simulink model "mrefrobotarm_previous_y_previous_u_previous_ref_cex_3b"  (R2018b)
settings: Solver=FixedStepAuto  StartTime=0.0  StopTime=20  RelTol=1e-3  AbsTol=1e-6
undefined symbols (not defined in the file or in its folder): cc, options
libraries: neural x462, simulink x2
(part 8 of 18)

== system mrefrobotarm_previous_y_previous_u_previous_ref_cex_3b/15000 epoch/Layer 3/Delays 1 ==
  "p{3}" : Inport  PortDimensions=30
      mask Display: e = 0.06;c1 = [120 230 180]/255;c2 = ([120 230 180]+0)/(256+128);c3 = ([120 230 180]+128)/(256+128);patch([0 1 1 0],[0 0 1 1],c1);patch([0 1 1 1-e 1-e 0+e],[0 0 1 1-e 0+e 0+e],c2);patch([0 0 1 1-e 0+e 0+e],[0 1 1 1-e 1-e 0+e],c3);plot([0 1 1 0 0],[0 0 1 1 0]);
  mux : Mux  Inputs=1
      mask Display: e = 0.06;c1 = [120 150 230]/255;c2 = ([120 150 230]+0)/383;c3 = ([120 150 230]+128)/383;patch([0 1 1 0],[0 0 1 1],c1);patch([0 1 1 1-e 1-e 0+e],[0 0 1 1-e 0+e 0+e],c2);patch([0 0 1 1-e 0+e 0+e],[0 1 1 1-e 1-e 0+e],c3);plot([0 1 1 0 0],[0 0 1 1 0]);disp('Mux')
  "pd{3,2}" : Outport
      mask Display: e = 0.06;c1 = [120 230 180]/255;c2 = ([120 230 180]+0)/(256+128);c3 = ([120 230 180]+128)/(256+128);patch([0 1 1 0],[0 0 1 1],c1);patch([0 1 1 1-e 1-e 0+e],[0 0 1 1-e 0+e 0+e],c2);patch([0 0 1 1-e 0+e 0+e],[0 1 1 1-e 1-e 0+e],c3);plot([0 1 1 0 0],[0 0 1 1 0]);
  wires:
  "p{3}"/1 -> mux/1
  mux/1 -> "pd{3,2}"/1

== system mrefrobotarm_previous_y_previous_u_previous_ref_cex_3b/15000 epoch/Layer 3/LW{3,2} ==
  "ad{3,2}" : Inport  PortDimensions=30
      mask Display: e = 0.06;c1 = [120 230 180]/255;c2 = ([120 230 180]+0)/(256+128);c3 = ([120 230 180]+128)/(256+128);patch([0 1 1 0],[0 0 1 1],c1);patch([0 1 1 1-e 1-e 0+e],[0 0 1 1-e 0+e 0+e],c2);patch([0 0 1 1-e 0+e 0+e],[0 1 1 1-e 1-e 0+e],c3);plot([0 1 1 0 0],[0 0 1 1 0]);
  "IW{3,2}(1,:)'" : Constant  Value=[0.85686770362183561910995877042296342551708221435546875;0.2506520137647199053532176549197174608707427978515625;0.5892150836046241568766390628297813236713409423828125;-0.7174409906013246018829931927029974758625030517578125;-0.68953568727712888364322907364112325012683868408203125;0.69140544006949611333112670763512142002582550048828125;0.5232408762883873354354591356241144239902496337890625;-0.087728735547543623685129432487883605062961578369140625;0.68082886601293768347176182942348532378673553466796875;-0.9464616786477015875078677709097974002361297607421875;-0.04449324205486195060732512729373411275446414947509765625;0.061158752469018307085235619524610228836536407470703125;0.08931518787288560135007031703935354016721248626708984375;-0.213826248773537452851911666584783233702182769775390625;-0.90148540581954550443555262972950004041194915771484375;-0.0972086798559116671558655298213125206530094146728515625;0.42254068930939803205859561785473488271236419677734375;0.1745984274977363526204499066807329654693603515625;-0.06359114155421728697969996346728294156491756439208984375;-0.35488973845845694921052881909417919814586639404296875;0.66414576011497239438341466666315682232379913330078125;0.81642799619769601537910830302280373871326446533203125;-0.1651023081874523901202422848655260168015956878662109375;0.5403352079923571249508995606447570025920867919921875;-0.286813174219213873339384690552833490073680877685546875;-0.09901539273150704312254077876787050627171993255615234375;0.5787096841793057944158817917923443019390106201171875;0.1940937926180541783782729226004448719322681427001953125;-0.52956768221008421182460779164102859795093536376953125;0.100064325977202328576964873718679882586002349853515625]
      mask Display: e = 0.06;c1 = [120 150 230]/255;c2 = ([120 150 230]+0)/383;c3 = ([120 150 230]+128)/383;patch([0 1 1 0],[0 0 1 1],c1);patch([0 1 1 1-e 1-e 0+e],[0 0 1 1-e 0+e 0+e],c2);patch([0 0 1 1-e 0+e 0+e],[0 1 1 1-e 1-e 0+e],c3);plot([0 1 1 0 0],[0 0 1 1 0]);disp('weights');
  Mux : Mux  Inputs=1
      mask Display: e = 0.06;c1 = [120 150 230]/255;c2 = ([120 150 230]+0)/383;c3 = ([120 150 230]+128)/383;patch([0 1 1 0],[0 0 1 1],c1);patch([0 1 1 1-e 1-e 0+e],[0 0 1 1-e 0+e 0+e],c2);patch([0 0 1 1-e 0+e 0+e],[0 1 1 1-e 1-e 0+e],c3);plot([0 1 1 0 0],[0 0 1 1 0]);disp('Mux');
  dotprod1 : neural/Weight Functions/dotprod
  "lz{3,2}" : Outport
      mask Display: e = 0.06;c1 = [120 230 180]/255;c2 = ([120 230 180]+0)/(256+128);c3 = ([120 230 180]+128)/(256+128);patch([0 1 1 0],[0 0 1 1],c1);patch([0 1 1 1-e 1-e 0+e],[0 0 1 1-e 0+e 0+e],c2);patch([0 0 1 1-e 0+e 0+e],[0 1 1 1-e 1-e 0+e],c3);plot([0 1 1 0 0],[0 0 1 1 0]);
  wires:
  "IW{3,2}(1,:)'"/1 -> dotprod1/1
  "ad{3,2}"/1 -> dotprod1/2
  dotprod1/1 -> Mux/1
  Mux/1 -> "lz{3,2}"/1

== system mrefrobotarm_previous_y_previous_u_previous_ref_cex_3b/5000_epoch/Layer 1/Delays 1 ==
  "p{1}" : Inport  PortDimensions=10
      mask Display: e = 0.06;c1 = [120 230 180]/255;c2 = ([120 230 180]+0)/(256+128);c3 = ([120 230 180]+128)/(256+128);patch([0 1 1 0],[0 0 1 1],c1);patch([0 1 1 1-e 1-e 0+e],[0 0 1 1-e 0+e 0+e],c2);patch([0 0 1 1-e 0+e 0+e],[0 1 1 1-e 1-e 0+e],c3);plot([0 1 1 0 0],[0 0 1 1 0]);
  mux : Mux  Inputs=1
      mask Display: e = 0.06;c1 = [120 150 230]/255;c2 = ([120 150 230]+0)/383;c3 = ([120 150 230]+128)/383;patch([0 1 1 0],[0 0 1 1],c1);patch([0 1 1 1-e 1-e 0+e],[0 0 1 1-e 0+e 0+e],c2);patch([0 0 1 1-e 0+e 0+e],[0 1 1 1-e 1-e 0+e],c3);plot([0 1 1 0 0],[0 0 1 1 0]);disp('Mux')
  "pd{1,1}" : Outport
      mask Display: e = 0.06;c1 = [120 230 180]/255;c2 = ([120 230 180]+0)/(256+128);c3 = ([120 230 180]+128)/(256+128);patch([0 1 1 0],[0 0 1 1],c1);patch([0 1 1 1-e 1-e 0+e],[0 0 1 1-e 0+e 0+e],c2);patch([0 0 1 1-e 0+e 0+e],[0 1 1 1-e 1-e 0+e],c3);plot([0 1 1 0 0],[0 0 1 1 0]);
  wires:
  "p{1}"/1 -> mux/1
  mux/1 -> "pd{1,1}"/1

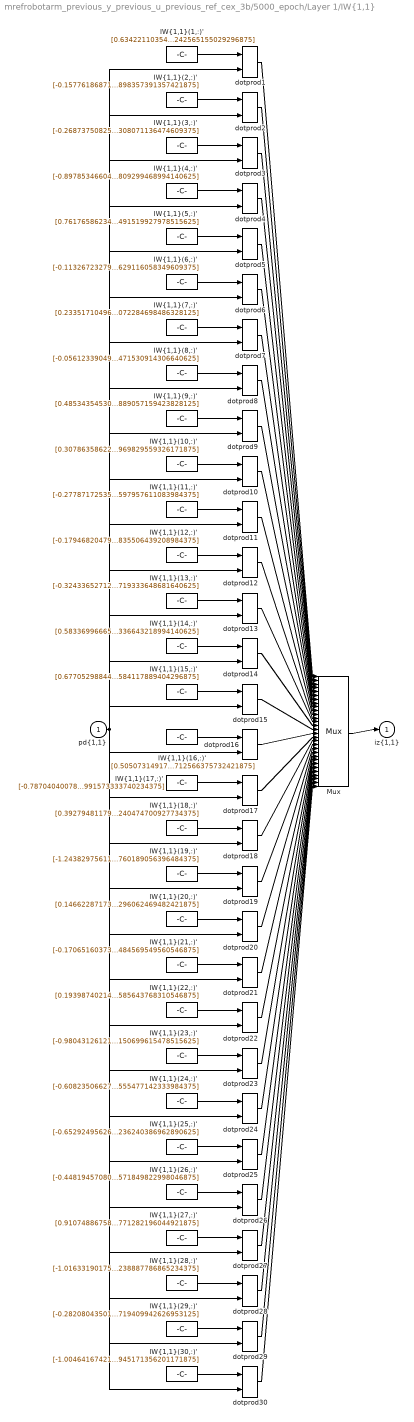
== system mrefrobotarm_previous_y_previous_u_previous_ref_cex_3b/5000_epoch/Layer 1/IW{1,1} ==
  "pd{1,1}" : Inport  PortDimensions=10
      mask Display: e = 0.06;c1 = [120 230 180]/255;c2 = ([120 230 180]+0)/(256+128);c3 = ([120 230 180]+128)/(256+128);patch([0 1 1 0],[0 0 1 1],c1);patch([0 1 1 1-e 1-e 0+e],[0 0 1 1-e 0+e 0+e],c2);patch([0 0 1 1-e 0+e 0+e],[0 1 1 1-e 1-e 0+e],c3);plot([0 1 1 0 0],[0 0 1 1 0]);
  "IW{1,1}(1,:)'" : Constant  Value=[0.63422110354193161896318997605703771114349365234375;-0.91869081932964802295060735559673048555850982666015625;0.59827755675717353422982114352635107934474945068359375;0.26110628531176161004623281769454479217529296875;-0.8543316435093497585029354013386182487010955810546875;-0.2051301151375984066493884938608971424400806427001953125;-0.9907677849565243999307995181879960000514984130859375;0.58997125932718319507586102190543897449970245361328125;0.2183879384389376399067117517915903590619564056396484375;-0.7436558763107175007434079816448502242565155029296875]
      mask Display: e = 0.06;c1 = [120 150 230]/255;c2 = ([120 150 230]+0)/383;c3 = ([120 150 230]+128)/383;patch([0 1 1 0],[0 0 1 1],c1);patch([0 1 1 1-e 1-e 0+e],[0 0 1 1-e 0+e 0+e],c2);patch([0 0 1 1-e 0+e 0+e],[0 1 1 1-e 1-e 0+e],c3);plot([0 1 1 0 0],[0 0 1 1 0]);disp('Weights');
  "IW{1,1}(10,:)'" : Constant  Value=[0.307863586226802266043733879996580071747303009033203125;0.665823350549687109634078296949155628681182861328125;-0.347044761319825256773441424229531548917293548583984375;-0.5363781767030550984287629034952260553836822509765625;1.050560745683177810150255027110688388347625732421875;0.0244046417058018418055898024476846330799162387847900390625;0.2430511761497498868234146129907458089292049407958984375;0.7826092295812963062218159393523819744586944580078125;-0.368356851635025517310850773355923593044281005859375;0.1818873004639951218575077973582665435969829559326171875]
      mask Display: e = 0.06;c1 = [120 150 230]/255;c2 = ([120 150 230]+0)/383;c3 = ([120 150 230]+128)/383;patch([0 1 1 0],[0 0 1 1],c1);patch([0 1 1 1-e 1-e 0+e],[0 0 1 1-e 0+e 0+e],c2);patch([0 0 1 1-e 0+e 0+e],[0 1 1 1-e 1-e 0+e],c3);plot([0 1 1 0 0],[0 0 1 1 0]);disp('Weights');
  "IW{1,1}(11,:)'" : Constant  Value=[-0.277871725357399956823911679748562164604663848876953125;0.727085385055948218990806708461605012416839599609375;-0.4177634282963211820316473676939494907855987548828125;0.35127268115717258378793985684751532971858978271484375;0.60674126246762305481041721577639691531658172607421875;0.262151794542885008265642454716726206243038177490234375;-0.32884797825156919515166009659878909587860107421875;1.228947726319721045484811838832683861255645751953125;-0.1372639006968274788533790342626161873340606689453125;0.3621595462750606397861474761157296597957611083984375]
      mask Display: e = 0.06;c1 = [120 150 230]/255;c2 = ([120 150 230]+0)/383;c3 = ([120 150 230]+128)/383;patch([0 1 1 0],[0 0 1 1],c1);patch([0 1 1 1-e 1-e 0+e],[0 0 1 1-e 0+e 0+e],c2);patch([0 0 1 1-e 0+e 0+e],[0 1 1 1-e 1-e 0+e],c3);plot([0 1 1 0 0],[0 0 1 1 0]);disp('Weights');
  "IW{1,1}(12,:)'" : Constant  Value=[-0.17946820479450542595856177285895682871341705322265625;0.0860802503761503301493718254278064705431461334228515625;1.0484706482704149177465069442405365407466888427734375;-1.0905649971679538534630182766704820096492767333984375;0.491324340439590556695037548706750385463237762451171875;0.02823068893210013696748461597962887026369571685791015625;0.3611184369846751618382540982565842568874359130859375;-0.346740473791346648368971727904863655567169189453125;0.49928270081376202593759217052138410508632659912109375;0.989842171249962543555511729209683835506439208984375]
      mask Display: e = 0.06;c1 = [120 150 230]/255;c2 = ([120 150 230]+0)/383;c3 = ([120 150 230]+128)/383;patch([0 1 1 0],[0 0 1 1],c1);patch([0 1 1 1-e 1-e 0+e],[0 0 1 1-e 0+e 0+e],c2);patch([0 0 1 1-e 0+e 0+e],[0 1 1 1-e 1-e 0+e],c3);plot([0 1 1 0 0],[0 0 1 1 0]);disp('Weights');
  "IW{1,1}(13,:)'" : Constant  Value=[-0.32433652712470062429161998807103373110294342041015625;-0.284421192666578281915690240566618740558624267578125;-2.012159445304701588241869103512726724147796630859375;0.9116130459235218808089484809897840023040771484375;0.7717671849933587235881304877693764865398406982421875;-0.85651593556354510550221448283991776406764984130859375;-1.22777179870519859150590491481125354766845703125;0.66179660226162451142073450682801194489002227783203125;0.066026002994952204261380757088772952556610107421875;1.956616810162020048124986715265549719333648681640625]
      mask Display: e = 0.06;c1 = [120 150 230]/255;c2 = ([120 150 230]+0)/383;c3 = ([120 150 230]+128)/383;patch([0 1 1 0],[0 0 1 1],c1);patch([0 1 1 1-e 1-e 0+e],[0 0 1 1-e 0+e 0+e],c2);patch([0 0 1 1-e 0+e 0+e],[0 1 1 1-e 1-e 0+e],c3);plot([0 1 1 0 0],[0 0 1 1 0]);disp('Weights');
  "IW{1,1}(14,:)'" : Constant  Value=[0.58336996665383178406472097776713781058788299560546875;0.322648507963840314172188072916469536721706390380859375;0.523765609130848464047858215053565800189971923828125;0.8058593121740205145187019297736696898937225341796875;-0.5143329303219184023276966399862430989742279052734375;0.9602600602832025433741591768921352922916412353515625;-0.97156821292382844479362802303512580692768096923828125;0.55408934836450907113203356857411563396453857421875;0.4215063659489122205314970415201969444751739501953125;4.34978727359094197169042672612704336643218994140625]
      mask Display: e = 0.06;c1 = [120 150 230]/255;c2 = ([120 150 230]+0)/383;c3 = ([120 150 230]+128)/383;patch([0 1 1 0],[0 0 1 1],c1);patch([0 1 1 1-e 1-e 0+e],[0 0 1 1-e 0+e 0+e],c2);patch([0 0 1 1-e 0+e 0+e],[0 1 1 1-e 1-e 0+e],c3);plot([0 1 1 0 0],[0 0 1 1 0]);disp('Weights');
  "IW{1,1}(15,:)'" : Constant  Value=[0.6770529884448668322960429577506147325038909912109375;-0.1553339993409601216267645895641180686652660369873046875;-2.59930933176377720883465372025966644287109375;-2.662436417357211926315585515112616121768951416015625;0.8357943645285363931662914183107204735279083251953125;0.428720996010904020767640076883253641426563262939453125;-0.421022258844727215176817480823956429958343505859375;-0.021294468736502140948640970918859238736331462860107421875;-0.67045413785377105941876152428449131548404693603515625;-0.833696285992292285271787477540783584117889404296875]
      mask Display: e = 0.06;c1 = [120 150 230]/255;c2 = ([120 150 230]+0)/383;c3 = ([120 150 230]+128)/383;patch([0 1 1 0],[0 0 1 1],c1);patch([0 1 1 1-e 1-e 0+e],[0 0 1 1-e 0+e 0+e],c2);patch([0 0 1 1-e 0+e 0+e],[0 1 1 1-e 1-e 0+e],c3);plot([0 1 1 0 0],[0 0 1 1 0]);disp('Weights');
  "IW{1,1}(16,:)'" : Constant  Value=[0.50507314917425538691730935170198790729045867919921875;5.816928027961356661990066641010344028472900390625;1.4256182078327797047023750565131194889545440673828125;-3.40685824055545793953569955192506313323974609375;1.1737201237286754018640522190253250300884246826171875;0.305003794417189499910136873950250446796417236328125;5.401774618303580410838549141772091388702392578125;-6.8709568655651640511905497987754642963409423828125;-5.87138509786090612152520407107658684253692626953125;4.42883250455615051777158441836945712566375732421875]
      mask Display: e = 0.06;c1 = [120 150 230]/255;c2 = ([120 150 230]+0)/383;c3 = ([120 150 230]+128)/383;patch([0 1 1 0],[0 0 1 1],c1);patch([0 1 1 1-e 1-e 0+e],[0 0 1 1-e 0+e 0+e],c2);patch([0 0 1 1-e 0+e 0+e],[0 1 1 1-e 1-e 0+e],c3);plot([0 1 1 0 0],[0 0 1 1 0]);disp('Weights');
  "IW{1,1}(17,:)'" : Constant  Value=[-0.78704040078131509705627877337974496185779571533203125;-1.134231229721498923623812515870667994022369384765625;-0.53361553923204085858600365099846385419368743896484375;0.32765683538617407233317635473213158547878265380859375;-0.07277466767389582924518975914907059632241725921630859375;0.050937769767023348410628358351459610275924205780029296875;0.316792128298135633457377480226568877696990966796875;0.8600335552910503000845210408442653715610504150390625;-0.2626194681353302140536243314272724092006683349609375;-0.061961761709411665444147132575380965135991573333740234375]
      mask Display: e = 0.06;c1 = [120 150 230]/255;c2 = ([120 150 230]+0)/383;c3 = ([120 150 230]+128)/383;patch([0 1 1 0],[0 0 1 1],c1);patch([0 1 1 1-e 1-e 0+e],[0 0 1 1-e 0+e 0+e],c2);patch([0 0 1 1-e 0+e 0+e],[0 1 1 1-e 1-e 0+e],c3);plot([0 1 1 0 0],[0 0 1 1 0]);disp('Weights');
  "IW{1,1}(18,:)'" : Constant  Value=[0.392794811797148535337242947207414545118808746337890625;0.307697573866610285531209001419483684003353118896484375;-0.047136023345347867474774972151863039471209049224853515625;-0.98539023410935067115445917806937359273433685302734375;-0.1839155396436170930574149906533421017229557037353515625;0.548927651149188733370465342886745929718017578125;-1.24965998951251844317766881431452929973602294921875;0.6145779349813675906943899462930858135223388671875;0.08348350800925861958656781780518940649926662445068359375;0.7475308837792675742406345307244919240474700927734375]
      mask Display: e = 0.06;c1 = [120 150 230]/255;c2 = ([120 150 230]+0)/383;c3 = ([120 150 230]+128)/383;patch([0 1 1 0],[0 0 1 1],c1);patch([0 1 1 1-e 1-e 0+e],[0 0 1 1-e 0+e 0+e],c2);patch([0 0 1 1-e 0+e 0+e],[0 1 1 1-e 1-e 0+e],c3);plot([0 1 1 0 0],[0 0 1 1 0]);disp('Weights');
  "IW{1,1}(19,:)'" : Constant  Value=[-1.24382975611538793003774117096327245235443115234375;-0.4632716178636535619972391941701062023639678955078125;0.253394080644103791843946282824617810547351837158203125;0.3106601850013317456244976710877381265163421630859375;-1.0483873203017106678913705763989128172397613525390625;-0.2671304450648310790938921854831278324127197265625;0.1879558132157162775310865754363476298749446868896484375;0.431489736241856658427451520765316672623157501220703125;0.730874589804547891702668493962846696376800537109375;1.0124736288655229454747086492716334760189056396484375]
      mask Display: e = 0.06;c1 = [120 150 230]/255;c2 = ([120 150 230]+0)/383;c3 = ([120 150 230]+128)/383;patch([0 1 1 0],[0 0 1 1],c1);patch([0 1 1 1-e 1-e 0+e],[0 0 1 1-e 0+e 0+e],c2);patch([0 0 1 1-e 0+e 0+e],[0 1 1 1-e 1-e 0+e],c3);plot([0 1 1 0 0],[0 0 1 1 0]);disp('Weights');
  "IW{1,1}(2,:)'" : Constant  Value=[-0.1577618687141210951363490266885492019355297088623046875;-0.91273360765273670036634712232626043260097503662109375;-0.6848523479687622650402545332326553761959075927734375;-1.041703036034508311757917908835224807262420654296875;-0.814000083702796306539539727964438498020172119140625;-0.266613983803191290089529275064705871045589447021484375;-0.3289343063292304858435954884043894708156585693359375;-0.291888983552204217541969910598709248006343841552734375;-0.433251183719709775932216189175960607826709747314453125;1.319568874721380069559018011204898357391357421875]
      mask Display: e = 0.06;c1 = [120 150 230]/255;c2 = ([120 150 230]+0)/383;c3 = ([120 150 230]+128)/383;patch([0 1 1 0],[0 0 1 1],c1);patch([0 1 1 1-e 1-e 0+e],[0 0 1 1-e 0+e 0+e],c2);patch([0 0 1 1-e 0+e 0+e],[0 1 1 1-e 1-e 0+e],c3);plot([0 1 1 0 0],[0 0 1 1 0]);disp('Weights');
  "IW{1,1}(20,:)'" : Constant  Value=[0.1466228717388136926214059485573670826852321624755859375;1.0330122936866847904724409090704284608364105224609375;-0.205801108223382323014760686419322155416011810302734375;0.83172979051121675997393367651966400444507598876953125;-0.466786454384762128366759270647889934480190277099609375;0.30474831700810367518528209984651766717433929443359375;0.87953900065965207044627049981500022113323211669921875;0.719108952043621574290455100708641111850738525390625;0.5757243754809648894621432191343046724796295166015625;-0.1984170060670278068482019762086565606296062469482421875]
      mask Display: e = 0.06;c1 = [120 150 230]/255;c2 = ([120 150 230]+0)/383;c3 = ([120 150 230]+128)/383;patch([0 1 1 0],[0 0 1 1],c1);patch([0 1 1 1-e 1-e 0+e],[0 0 1 1-e 0+e 0+e],c2);patch([0 0 1 1-e 0+e 0+e],[0 1 1 1-e 1-e 0+e],c3);plot([0 1 1 0 0],[0 0 1 1 0]);disp('Weights');
  "IW{1,1}(21,:)'" : Constant  Value=[-0.1706516037301274713033905072734341956675052642822265625;0.2552832032408678397672474602586589753627777099609375;-0.9970359897900216150645746893133036792278289794921875;-0.50311319744039473267349649177049286663532257080078125;-0.851031526737401566862217805464752018451690673828125;-0.301019200262316710681176346042775548994541168212890625;0.58888125984900263620858140711789019405841827392578125;0.4922378060099343866085064291837625205516815185546875;-0.1740697076945744437015406447244458831846714019775390625;1.109311081835623991054262660327367484569549560546875]
      mask Display: e = 0.06;c1 = [120 150 230]/255;c2 = ([120 150 230]+0)/383;c3 = ([120 150 230]+128)/383;patch([0 1 1 0],[0 0 1 1],c1);patch([0 1 1 1-e 1-e 0+e],[0 0 1 1-e 0+e 0+e],c2);patch([0 0 1 1-e 0+e 0+e],[0 1 1 1-e 1-e 0+e],c3);plot([0 1 1 0 0],[0 0 1 1 0]);disp('Weights');
  "IW{1,1}(22,:)'" : Constant  Value=[0.193987402143908027607466237896005623042583465576171875;1.0977355379300346438498081624857150018215179443359375;-0.39691028812462791908188819434144534170627593994140625;-0.379708152173499013937174595412216149270534515380859375;-0.7972368630469872652355434183846227824687957763671875;0.80429873483767122532839266568771563470363616943359375;-0.3496472305647546630069655293482355773448944091796875;-0.28629504686716844563676431789644993841648101806640625;0.0833025836648184359045643532226677052676677703857421875;-0.87067519420473427071982541747274808585643768310546875]
      mask Display: e = 0.06;c1 = [120 150 230]/255;c2 = ([120 150 230]+0)/383;c3 = ([120 150 230]+128)/383;patch([0 1 1 0],[0 0 1 1],c1);patch([0 1 1 1-e 1-e 0+e],[0 0 1 1-e 0+e 0+e],c2);patch([0 0 1 1-e 0+e 0+e],[0 1 1 1-e 1-e 0+e],c3);plot([0 1 1 0 0],[0 0 1 1 0]);disp('Weights');
  "IW{1,1}(23,:)'" : Constant  Value=[-0.98043126121720425292238587644533254206180572509765625;0.5187162040008452823514062401955015957355499267578125;0.09493691627132662402832607995151192881166934967041015625;-1.2792813524514803358300696345395408570766448974609375;1.826601613423700865013188376906327903270721435546875;-1.1270284416244502612158839838230051100254058837890625;0.031961501789579425947263047191881923936307430267333984375;-0.334719557619565788453286359072080813348293304443359375;-0.097824781976371066871678294774028472602367401123046875;-0.51973005675672911962692523957230150699615478515625]
      mask Display: e = 0.06;c1 = [120 150 230]/255;c2 = ([120 150 230]+0)/383;c3 = ([120 150 230]+128)/383;patch([0 1 1 0],[0 0 1 1],c1);patch([0 1 1 1-e 1-e 0+e],[0 0 1 1-e 0+e 0+e],c2);patch([0 0 1 1-e 0+e 0+e],[0 1 1 1-e 1-e 0+e],c3);plot([0 1 1 0 0],[0 0 1 1 0]);disp('Weights');
  "IW{1,1}(24,:)'" : Constant  Value=[-0.60823506627433598925591695660841651260852813720703125;-1.0350954638719700451332528245984576642513275146484375;0.388403799366780766444406935988808982074260711669921875;0.414541347441563401421404932989389635622501373291015625;0.1530538176110360082393668790246010757982730865478515625;-0.6507114418750361561905037888209335505962371826171875;-1.0530908168736445862379014215548522770404815673828125;-0.63920610168342240076100324586150236427783966064453125;0.07720915498782608687999839958138181827962398529052734375;-1.2792376146281101423340942346840165555477142333984375]
      mask Display: e = 0.06;c1 = [120 150 230]/255;c2 = ([120 150 230]+0)/383;c3 = ([120 150 230]+128)/383;patch([0 1 1 0],[0 0 1 1],c1);patch([0 1 1 1-e 1-e 0+e],[0 0 1 1-e 0+e 0+e],c2);patch([0 0 1 1-e 0+e 0+e],[0 1 1 1-e 1-e 0+e],c3);plot([0 1 1 0 0],[0 0 1 1 0]);disp('Weights');
  "IW{1,1}(25,:)'" : Constant  Value=[-0.652924956262813882545970045612193644046783447265625;0.80432253900291750259299305980675853788852691650390625;-0.025138027958748775103625661131445667706429958343505859375;-0.59292425073382004629962693798006512224674224853515625;-0.8006524348822920966739502546261064708232879638671875;-0.75205906006257505769241333837271668016910552978515625;-0.60629551488591382213400038381223566830158233642578125;0.7533263406753050173136898592929355800151824951171875;-0.33714285136075605731065252257394604384899139404296875;1.336484316350615930701906108879484236240386962890625]
      mask Display: e = 0.06;c1 = [120 150 230]/255;c2 = ([120 150 230]+0)/383;c3 = ([120 150 230]+128)/383;patch([0 1 1 0],[0 0 1 1],c1);patch([0 1 1 1-e 1-e 0+e],[0 0 1 1-e 0+e 0+e],c2);patch([0 0 1 1-e 0+e 0+e],[0 1 1 1-e 1-e 0+e],c3);plot([0 1 1 0 0],[0 0 1 1 0]);disp('Weights');
  "IW{1,1}(26,:)'" : Constant  Value=[-0.448194570807548486879312577002565376460552215576171875;-1.05590877664238913524741292349062860012054443359375;-0.55381010671810348977572857620543800294399261474609375;0.273047258128943204358307639267877675592899322509765625;0.68393789685749772910838828465784899890422821044921875;-0.552049634459655269580480307922698557376861572265625;-0.71179782246324341254961609593010507524013519287109375;-0.6213625047085991059958587356959469616413116455078125;1.111446504428653891949352328083477914333343505859375;-0.436355183585302508486591932523879222571849822998046875]
      mask Display: e = 0.06;c1 = [120 150 230]/255;c2 = ([120 150 230]+0)/383;c3 = ([120 150 230]+128)/383;patch([0 1 1 0],[0 0 1 1],c1);patch([0 1 1 1-e 1-e 0+e],[0 0 1 1-e 0+e 0+e],c2);patch([0 0 1 1-e 0+e 0+e],[0 1 1 1-e 1-e 0+e],c3);plot([0 1 1 0 0],[0 0 1 1 0]);disp('Weights');
  "IW{1,1}(27,:)'" : Constant  Value=[0.91074886758763951011275139535428024828433990478515625;-0.7601629699673464468645533997914753854274749755859375;0.61207093811119561710398784271092154085636138916015625;-0.5478044094258915919226637925021350383758544921875;0.40158232560320528126140970925916917622089385986328125;0.52009915573271559008361464293557219207286834716796875;-0.18081440484775923582816403722972609102725982666015625;-0.329871448172018910671710045789950527250766754150390625;-1.138553856823875332082707245717756450176239013671875;0.318521333708069398493734070143545977771282196044921875]
      mask Display: e = 0.06;c1 = [120 150 230]/255;c2 = ([120 150 230]+0)/383;c3 = ([120 150 230]+128)/383;patch([0 1 1 0],[0 0 1 1],c1);patch([0 1 1 1-e 1-e 0+e],[0 0 1 1-e 0+e 0+e],c2);patch([0 0 1 1-e 0+e 0+e],[0 1 1 1-e 1-e 0+e],c3);plot([0 1 1 0 0],[0 0 1 1 0]);disp('Weights');
  "IW{1,1}(28,:)'" : Constant  Value=[-1.01633190175224452644897610298357903957366943359375;-0.73465882460576537038576816485146991908550262451171875;-0.35171298148601304323079830282949842512607574462890625;0.53014538696878965584602383387391455471515655517578125;0.6646965210807582735696996678598225116729736328125;0.2491060258368409663365383721611578948795795440673828125;-0.79108705496805009627081517464830540120601654052734375;0.30173326377861808822444800171069800853729248046875;0.2496703363633840933033525288919918239116668701171875;-0.77150607535184556606822070534690283238887786865234375]
      mask Display: e = 0.06;c1 = [120 150 230]/255;c2 = ([120 150 230]+0)/383;c3 = ([120 150 230]+128)/383;patch([0 1 1 0],[0 0 1 1],c1);patch([0 1 1 1-e 1-e 0+e],[0 0 1 1-e 0+e 0+e],c2);patch([0 0 1 1-e 0+e 0+e],[0 1 1 1-e 1-e 0+e],c3);plot([0 1 1 0 0],[0 0 1 1 0]);disp('Weights');
  "IW{1,1}(29,:)'" : Constant  Value=[-0.2820804350125569737173236717353574931621551513671875;1.119305584191458979859135070000775158405303955078125;0.56980276284833120126194216936710290610790252685546875;0.55639258172968608651132171871722675859928131103515625;0.79202180324043636172604010425857268273830413818359375;0.349457599732402035552780716898269020020961761474609375;-0.180836356813649345998129547297139652073383331298828125;-1.2307004599689383983474044725880958139896392822265625;1.65388306443919308463819106691516935825347900390625;0.0475949606288715021396029669631388969719409942626953125]
      mask Display: e = 0.06;c1 = [120 150 230]/255;c2 = ([120 150 230]+0)/383;c3 = ([120 150 230]+128)/383;patch([0 1 1 0],[0 0 1 1],c1);patch([0 1 1 1-e 1-e 0+e],[0 0 1 1-e 0+e 0+e],c2);patch([0 0 1 1-e 0+e 0+e],[0 1 1 1-e 1-e 0+e],c3);plot([0 1 1 0 0],[0 0 1 1 0]);disp('Weights');
  "IW{1,1}(3,:)'" : Constant  Value=[-0.268737508256914114923574743443168699741363525390625;-0.25042137066598957328977803626912645995616912841796875;0.4880422237661969919741977719240821897983551025390625;0.24011704503183606274063777163974009454250335693359375;1.1638401758862653156967326140147633850574493408203125;-0.5966688691768966545936336842714808881282806396484375;-0.53958677542689503781048188102431595325469970703125;1.0104963610440613752672334157978184521198272705078125;9.983163741769214283294786582700908184051513671875;1.4233456246584841320412806453532539308071136474609375]
      mask Display: e = 0.06;c1 = [120 150 230]/255;c2 = ([120 150 230]+0)/383;c3 = ([120 150 230]+128)/383;patch([0 1 1 0],[0 0 1 1],c1);patch([0 1 1 1-e 1-e 0+e],[0 0 1 1-e 0+e 0+e],c2);patch([0 0 1 1-e 0+e 0+e],[0 1 1 1-e 1-e 0+e],c3);plot([0 1 1 0 0],[0 0 1 1 0]);disp('Weights');
  "IW{1,1}(30,:)'" : Constant  Value=[-1.0046416742164769875245156072196550667285919189453125;0.429749853528365033383806803612969815731048583984375;-0.63671674477197293118280185808544047176837921142578125;0.464500286896545155901350199201260693371295928955078125;-0.08323146695230380920360602203800226561725139617919921875;0.97772984948489527479154048705822788178920745849609375;-0.82934845336514040337050346352043561637401580810546875;0.152758873586543997280529083582223393023014068603515625;0.08535591138308830372327662416864768601953983306884765625;0.77639828376222552730467896253685466945171356201171875]
      mask Display: e = 0.06;c1 = [120 150 230]/255;c2 = ([120 150 230]+0)/383;c3 = ([120 150 230]+128)/383;patch([0 1 1 0],[0 0 1 1],c1);patch([0 1 1 1-e 1-e 0+e],[0 0 1 1-e 0+e 0+e],c2);patch([0 0 1 1-e 0+e 0+e],[0 1 1 1-e 1-e 0+e],c3);plot([0 1 1 0 0],[0 0 1 1 0]);disp('Weights');
  "IW{1,1}(4,:)'" : Constant  Value=[-0.89785346604696558703295750092365778982639312744140625;-0.41486643533670031214199980240664444863796234130859375;-4.30730761802675488070235587656497955322265625;0.92877315210754984864394145915866829454898834228515625;-0.486976161928859452299178656176081858575344085693359375;-0.6507393119280016069438943304703570902347564697265625;0.647102972530151365759820691891945898532867431640625;-0.86912858004302229186777140057529322803020477294921875;13.1875881727896508976982659078203141689300537109375;-7.77104830476519570225946154096163809299468994140625]
      mask Display: e = 0.06;c1 = [120 150 230]/255;c2 = ([120 150 230]+0)/383;c3 = ([120 150 230]+128)/383;patch([0 1 1 0],[0 0 1 1],c1);patch([0 1 1 1-e 1-e 0+e],[0 0 1 1-e 0+e 0+e],c2);patch([0 0 1 1-e 0+e 0+e],[0 1 1 1-e 1-e 0+e],c3);plot([0 1 1 0 0],[0 0 1 1 0]);disp('Weights');
  "IW{1,1}(5,:)'" : Constant  Value=[0.7617658623438814391448659080197103321552276611328125;0.697116937645829271019692896516062319278717041015625;-1.0429794333165685049635840186965651810169219970703125;-0.11879079310224949228569357728702016174793243408203125;0.175616731935968939382064490928314626216888427734375;-0.1504976558881047921101270503640989772975444793701171875;0.38681395529327755600235150268417783081531524658203125;0.013430254728329878155523857685693656094372272491455078125;-1.135835416271210096539334699627943336963653564453125;0.1208944257977057346042926155860186554491519927978515625]
      mask Display: e = 0.06;c1 = [120 150 230]/255;c2 = ([120 150 230]+0)/383;c3 = ([120 150 230]+128)/383;patch([0 1 1 0],[0 0 1 1],c1);patch([0 1 1 1-e 1-e 0+e],[0 0 1 1-e 0+e 0+e],c2);patch([0 0 1 1-e 0+e 0+e],[0 1 1 1-e 1-e 0+e],c3);plot([0 1 1 0 0],[0 0 1 1 0]);disp('Weights');
  "IW{1,1}(6,:)'" : Constant  Value=[-0.11326723279748852901693823014284134842455387115478515625;1.1567450115129880305886445057694800198078155517578125;0.048525646477535676337478065534014604054391384124755859375;0.85424860003408209507824722095392644405364990234375;0.1343131846707333043600129940386977978050708770751953125;0.54468608453891886878039940711460076272487640380859375;-0.465523672464658921921198952986742369830608367919921875;-0.03837361732594136987106736569330678321421146392822265625;-0.64043551527332154282845522175193764269351959228515625;-0.3778927548269341851749913985258899629116058349609375]
      mask Display: e = 0.06;c1 = [120 150 230]/255;c2 = ([120 150 230]+0)/383;c3 = ([120 150 230]+128)/383;patch([0 1 1 0],[0 0 1 1],c1);patch([0 1 1 1-e 1-e 0+e],[0 0 1 1-e 0+e 0+e],c2);patch([0 0 1 1-e 0+e 0+e],[0 1 1 1-e 1-e 0+e],c3);plot([0 1 1 0 0],[0 0 1 1 0]);disp('Weights');
  "IW{1,1}(7,:)'" : Constant  Value=[0.2335171049668950671307499078466207720339298248291015625;2.481271126467852194963370493496768176555633544921875;-0.5791835349983542879925835222820751368999481201171875;-0.91262122382761201588863286815467290580272674560546875;1.7539788749764344544246341683901846408843994140625;0.15446164078708590761124241907964460551738739013671875;-1.6752904191857849180991024695686064660549163818359375;-1.1953302193678478904104167668265290558338165283203125;0.1466345594694015985748336561300675384700298309326171875;-1.5591796195238487587886311303009279072284698486328125]
      mask Display: e = 0.06;c1 = [120 150 230]/255;c2 = ([120 150 230]+0)/383;c3 = ([120 150 230]+128)/383;patch([0 1 1 0],[0 0 1 1],c1);patch([0 1 1 1-e 1-e 0+e],[0 0 1 1-e 0+e 0+e],c2);patch([0 0 1 1-e 0+e 0+e],[0 1 1 1-e 1-e 0+e],c3);plot([0 1 1 0 0],[0 0 1 1 0]);disp('Weights');
  "IW{1,1}(8,:)'" : Constant  Value=[-0.05612339049880270269721194154044496826827526092529296875;0.17099533102751329760593534956569783389568328857421875;0.414501386745428301860982855941983871161937713623046875;-1.0812999136099421537693388017942197620868682861328125;0.93012406100425348842719586173188872635364532470703125;1.123108017385306300894853848149068653583526611328125;-0.1740205823952052366365705893258564174175262451171875;0.5106076015383600452679502268438227474689483642578125;-1.9748988804559761689461083733476698398590087890625;-1.02915858210311572662476464756764471530914306640625]
      mask Display: e = 0.06;c1 = [120 150 230]/255;c2 = ([120 150 230]+0)/383;c3 = ([120 150 230]+128)/383;patch([0 1 1 0],[0 0 1 1],c1);patch([0 1 1 1-e 1-e 0+e],[0 0 1 1-e 0+e 0+e],c2);patch([0 0 1 1-e 0+e 0+e],[0 1 1 1-e 1-e 0+e],c3);plot([0 1 1 0 0],[0 0 1 1 0]);disp('Weights');
  "IW{1,1}(9,:)'" : Constant  Value=[0.485343545303149659364549961537704803049564361572265625;0.73269181354778412096351303262053988873958587646484375;0.494980882105890584998775239000678993761539459228515625;-0.73643466096360843398116458047297783195972442626953125;0.199864756436801294103844384153489954769611358642578125;0.50635823529042289781187946573481895029544830322265625;0.85703656273813788590842932535451836884021759033203125;0.691509109447839609430275231716223061084747314453125;-1.683838741554396722932551710982806980609893798828125;-1.672778919230424765629550165613181889057159423828125]
      mask Display: e = 0.06;c1 = [120 150 230]/255;c2 = ([120 150 230]+0)/383;c3 = ([120 150 230]+128)/383;patch([0 1 1 0],[0 0 1 1],c1);patch([0 1 1 1-e 1-e 0+e],[0 0 1 1-e 0+e 0+e],c2);patch([0 0 1 1-e 0+e 0+e],[0 1 1 1-e 1-e 0+e],c3);plot([0 1 1 0 0],[0 0 1 1 0]);disp('Weights');
  Mux : Mux  Inputs=30
      mask Display: e = 0.06;c1 = [120 150 230]/255;c2 = ([120 150 230]+0)/383;c3 = ([120 150 230]+128)/383;patch([0 1 1 0],[0 0 1 1],c1);patch([0 1 1 1-e 1-e 0+e],[0 0 1 1-e 0+e 0+e],c2);patch([0 0 1 1-e 0+e 0+e],[0 1 1 1-e 1-e 0+e],c3);plot([0 1 1 0 0],[0 0 1 1 0]);disp('Mux');
  dotprod{1..30} (30 alike) : neural/Weight Functions/dotprod
  "iz{1,1}" : Outport
      mask Display: e = 0.06;c1 = [120 230 180]/255;c2 = ([120 230 180]+0)/(256+128);c3 = ([120 230 180]+128)/(256+128);patch([0 1 1 0],[0 0 1 1],c1);patch([0 1 1 1-e 1-e 0+e],[0 0 1 1-e 0+e 0+e],c2);patch([0 0 1 1-e 0+e 0+e],[0 1 1 1-e 1-e 0+e],c3);plot([0 1 1 0 0],[0 0 1 1 0]);
  wires:
  "IW{1,1}(1,:)'"/1 -> dotprod1/1
  "pd{1,1}"/1 -> dotprod1/2, dotprod2/2, dotprod3/2, dotprod4/2, dotprod5/2, dotprod6/2, dotprod7/2, dotprod8/2, dotprod9/2, dotprod10/2, dotprod11/2, dotprod12/2, dotprod13/2, dotprod14/2, dotprod15/2, dotprod16/2, dotprod17/2, dotprod18/2, dotprod19/2, dotprod20/2, dotprod21/2, dotprod22/2, dotprod23/2, dotprod24/2, dotprod25/2, dotprod26/2, dotprod27/2, dotprod28/2, dotprod29/2, dotprod30/2
  dotprod1/1 -> Mux/1
  "IW{1,1}(2,:)'"/1 -> dotprod2/1
  dotprod2/1 -> Mux/2
  "IW{1,1}(3,:)'"/1 -> dotprod3/1
  dotprod3/1 -> Mux/3
  "IW{1,1}(4,:)'"/1 -> dotprod4/1
  dotprod4/1 -> Mux/4
  "IW{1,1}(5,:)'"/1 -> dotprod5/1
  dotprod5/1 -> Mux/5
  "IW{1,1}(6,:)'"/1 -> dotprod6/1
  dotprod6/1 -> Mux/6
  "IW{1,1}(7,:)'"/1 -> dotprod7/1
  dotprod7/1 -> Mux/7
  "IW{1,1}(8,:)'"/1 -> dotprod8/1
  dotprod8/1 -> Mux/8
  "IW{1,1}(9,:)'"/1 -> dotprod9/1
  dotprod9/1 -> Mux/9
  "IW{1,1}(10,:)'"/1 -> dotprod10/1
  dotprod10/1 -> Mux/10
  "IW{1,1}(11,:)'"/1 -> dotprod11/1
  dotprod11/1 -> Mux/11
  "IW{1,1}(12,:)'"/1 -> dotprod12/1
  dotprod12/1 -> Mux/12
  "IW{1,1}(13,:)'"/1 -> dotprod13/1
  dotprod13/1 -> Mux/13
  "IW{1,1}(14,:)'"/1 -> dotprod14/1
  dotprod14/1 -> Mux/14
  "IW{1,1}(15,:)'"/1 -> dotprod15/1
  dotprod15/1 -> Mux/15
  "IW{1,1}(16,:)'"/1 -> dotprod16/1
  dotprod16/1 -> Mux/16
  "IW{1,1}(17,:)'"/1 -> dotprod17/1
  dotprod17/1 -> Mux/17
  "IW{1,1}(18,:)'"/1 -> dotprod18/1
  dotprod18/1 -> Mux/18
  "IW{1,1}(19,:)'"/1 -> dotprod19/1
  dotprod19/1 -> Mux/19
  "IW{1,1}(20,:)'"/1 -> dotprod20/1
  dotprod20/1 -> Mux/20
  "IW{1,1}(21,:)'"/1 -> dotprod21/1
  dotprod21/1 -> Mux/21
  "IW{1,1}(22,:)'"/1 -> dotprod22/1
  dotprod22/1 -> Mux/22
  "IW{1,1}(23,:)'"/1 -> dotprod23/1
  dotprod23/1 -> Mux/23
  "IW{1,1}(24,:)'"/1 -> dotprod24/1
  dotprod24/1 -> Mux/24
  "IW{1,1}(25,:)'"/1 -> dotprod25/1
  dotprod25/1 -> Mux/25
  "IW{1,1}(26,:)'"/1 -> dotprod26/1
  dotprod26/1 -> Mux/26
  "IW{1,1}(27,:)'"/1 -> dotprod27/1
  dotprod27/1 -> Mux/27
  "IW{1,1}(28,:)'"/1 -> dotprod28/1
  dotprod28/1 -> Mux/28
  "IW{1,1}(29,:)'"/1 -> dotprod29/1
  dotprod29/1 -> Mux/29
  "IW{1,1}(30,:)'"/1 -> dotprod30/1
  dotprod30/1 -> Mux/30
  Mux/1 -> "iz{1,1}"/1

== system mrefrobotarm_previous_y_previous_u_previous_ref_cex_3b/5000_epoch/Layer 2/Delays 1 ==
  "p{2}" : Inport  PortDimensions=30
      mask Display: e = 0.06;c1 = [120 230 180]/255;c2 = ([120 230 180]+0)/(256+128);c3 = ([120 230 180]+128)/(256+128);patch([0 1 1 0],[0 0 1 1],c1);patch([0 1 1 1-e 1-e 0+e],[0 0 1 1-e 0+e 0+e],c2);patch([0 0 1 1-e 0+e 0+e],[0 1 1 1-e 1-e 0+e],c3);plot([0 1 1 0 0],[0 0 1 1 0]);
  mux : Mux  Inputs=1
      mask Display: e = 0.06;c1 = [120 150 230]/255;c2 = ([120 150 230]+0)/383;c3 = ([120 150 230]+128)/383;patch([0 1 1 0],[0 0 1 1],c1);patch([0 1 1 1-e 1-e 0+e],[0 0 1 1-e 0+e 0+e],c2);patch([0 0 1 1-e 0+e 0+e],[0 1 1 1-e 1-e 0+e],c3);plot([0 1 1 0 0],[0 0 1 1 0]);disp('Mux')
  "pd{2,1}" : Outport
      mask Display: e = 0.06;c1 = [120 230 180]/255;c2 = ([120 230 180]+0)/(256+128);c3 = ([120 230 180]+128)/(256+128);patch([0 1 1 0],[0 0 1 1],c1);patch([0 1 1 1-e 1-e 0+e],[0 0 1 1-e 0+e 0+e],c2);patch([0 0 1 1-e 0+e 0+e],[0 1 1 1-e 1-e 0+e],c3);plot([0 1 1 0 0],[0 0 1 1 0]);
  wires:
  "p{2}"/1 -> mux/1
  mux/1 -> "pd{2,1}"/1
